simulink model "Navigation_Simple"  (R2016b)
settings: Solver=VariableStepAuto  StartTime=0.0  StopTime=10.0  RelTol=1e-3
values from neighbouring files (symbols this model uses):
  Env =     [UAV_modelconfig.mat]
  TrimCondition =     [UAV_trimcondition.mat]
libraries: Navigation_Lib x3
settings Model: Creator=UAVLAB  LastModifiedBy=UAVLAB

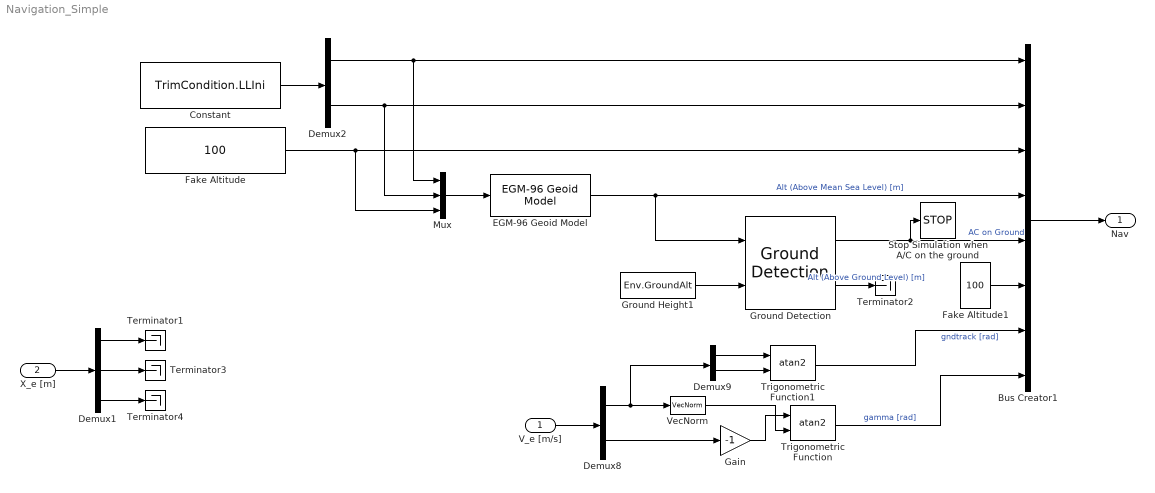
== system Navigation_Simple ==
  V_e [m/s] : Inport
  X_e [m] : Inport  Port=2
  Bus Creator1 : BusCreator  Inputs=8  OutDataTypeStr=Bus: Nav
      settings: InheritFromInputs=off
  Constant : Constant  Value=TrimCondition.LLIni
  Demux1 : Demux  Outputs=3
  Demux2 : Demux  Outputs=2
  Demux8 : Demux  Outputs=[2 1]
  Demux9 : Demux  Outputs=2
  EGM-96 Geoid Model : Navigation_Lib/Navigation/EGM-96 Geoid Model
  Fake Altitude : Constant  Value=100
  Fake Altitude1 : Constant  Value=100
  Gain : Gain  Gain=-1
  Ground Detection : Navigation_Lib/Navigation/Ground Detection
  Ground Height1 : Constant  Value=Env.GroundAlt
  Mux : Mux  Inputs=3
  Stop Simulation when A/C on the ground : Stop
  Terminator{1..4} (4 alike) : Terminator
  Trigonometric Function : Trigonometry  Operator=atan2
  Trigonometric Function1 : Trigonometry  Operator=atan2
  VecNorm : Navigation_Lib/Navigation/VecNorm
  Nav : Outport  OutDataTypeStr=Bus: Nav
  wires:
  Bus Creator1/1 -> Nav/1
  X_e [m]/1 -> Demux1/1
  Demux1/1 -> Terminator1/1
  Demux1/2 -> Terminator3/1
  Demux1/3 -> Terminator4/1
  Constant/1 -> Demux2/1
  Demux2/1 -> Mux/1, Bus Creator1/1
  Demux2/2 -> Mux/2, Bus Creator1/2
  EGM-96 Geoid Model/1 -> Ground Detection/1, Bus Creator1/4  "Alt (Above Mean Sea Level) [m]"
  Ground Height1/1 -> Ground Detection/2
  Ground Detection/1 -> Stop Simulation when A/C on the ground/1, Bus Creator1/5  "AC on Ground"
  V_e [m/s]/1 -> Demux8/1
  Demux8/2 -> Gain/1
  VecNorm/1 -> Trigonometric Function/2
  Trigonometric Function/1 -> Bus Creator1/8  "gamma [rad]"
  Demux9/2 -> Trigonometric Function1/2
  Trigonometric Function1/1 -> Bus Creator1/7  "gndtrack [rad]"
  Demux8/1 -> VecNorm/1, Demux9/1
  Demux9/1 -> Trigonometric Function1/1
  Gain/1 -> Trigonometric Function/1
  Fake Altitude/1 -> Mux/3, Bus Creator1/3
  Mux/1 -> EGM-96 Geoid Model/1
  Fake Altitude1/1 -> Bus Creator1/6
  Ground Detection/2 -> Terminator2/1  "Alt (Above Ground Level) [m]"
